simulink model "iface"  (R2018b)
settings: Solver=FixedStepDiscrete  StartTime=0.0  StopTime=10.0  RelTol=1e-3
settings Model: Creator=matlab  LastModifiedBy=matlab

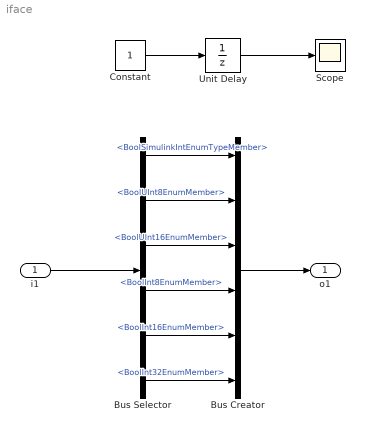
== system iface ==
  i1 : Inport  OutDataTypeStr=Bus: BusDef
  Bus Creator : BusCreator  Inputs=6  OutDataTypeStr=Bus: BusDef  NonVirtualBus=on
  Bus Selector : BusSelector  OutputSignals=BoolSimulinkIntEnumTypeMember,BoolUInt8EnumMember,BoolUInt16EnumMember,BoolInt8EnumMember,BoolInt16EnumMember,BoolInt32EnumMember
  Constant : Constant
  Scope : Scope
  Unit Delay : UnitDelay  SampleTime=-1
  o1 : Outport  OutDataTypeStr=Bus: BusDef
  wires:
  Bus Creator/1 -> o1/1
  i1/1 -> Bus Selector/1
  Unit Delay/1 -> Scope/1
  Constant/1 -> Unit Delay/1
  Bus Selector/1 -> Bus Creator/1  "<BoolSimulinkIntEnumTypeMember>"
  Bus Selector/2 -> Bus Creator/2  "<BoolUInt8EnumMember>"
  Bus Selector/3 -> Bus Creator/3  "<BoolUInt16EnumMember>"
  Bus Selector/4 -> Bus Creator/4  "<BoolInt8EnumMember>"
  Bus Selector/5 -> Bus Creator/5  "<BoolInt16EnumMember>"
  Bus Selector/6 -> Bus Creator/6  "<BoolInt32EnumMember>"
